simulink library "SUB_ECU_L4_MABX_HW_Interface"  (R2018a)
settings: Solver=VariableStepAuto  StartTime=0.0  StopTime=10.0  RelTol=1e-3
PostLoadFcn:
  | , if any(exist('dsrtsu_mdlpostloadfcn', 'file') == [2, 3, 6]), try dsrtsu_mdlpostloadfcn('Execute', bdroot); catch fprintf('Error in PostLoadFcn (dsrtsu_mdlpostloadfcn) for model "%s":\n %s\n', bdroot, lasterr); end, end,
undefined symbols (not defined in the file or in its folder): CANR_PROPB_REAX_3_13_CHANNEL_APV, CANR_PROPB_REAX_4_13_CHANNEL_APV, CANR_PROPB_XPR_1_50_CHANNEL_APV, ENUM_CAN_RX_T, ENUM_CAN_TX_T, ENUM_REAX_OPERATION_MODE_T, ENUM_SIGNAL_HEALTH_T, ENUM_XBR_CONTROL_MODE_T, ENUM_XBR_EBI_MODE_T, ENUM_XBR_PASS_THROUGH_ACTIVE_T, ENUM_XBR_PRIORITY_T, ENUM_XPR_INHIBIT_PARK_MANUAL_T, ENUM_XPR_INHIBIT_UNPARK_MANUAL_T, ENUM_XPR_PARK_MANUAL_T, ENUM_XPR_UNPARK_MANUAL_T, PROPB_REAX_1_E4_DES_POS_SIG_SRC_APV, PROPB_REAX_1_E4_DESIRED_OPMODE_APV, PROPB_REAX_1_E4_DESIRED_POSITION_APV, ptc_matlab_lib
libraries: PTC_MBDS_LIB x264, rtican x172, EmE_MBD_Blockset x39, simulink x34, $bdroot x16, rti1401lib_dio_type4 x8, simulink_need_slupdate x7, dsa_tcpip_lib x4, rti1401lib_adc_type4 x3, rtmapslib x3, rtitasklib x3
(part 45 of 51)

== system SUB_ECU_L4_MABX_HW_Interface/CAN_Out_PTC_1571/CAN_TX_1000ms/CAN_TX_AMB_00/TX_CAN4 ==
  Enable : Inport
  Data : Inport  Port=2
  AMB : rtican/RTICAN Transmit (TX)   Reserved1=[]  Reserved2=[]  Reserved3=[]  Reserved4=[]  SfcnMessage=[]  Msg_Struct=[]  BoardTypeNo=[]  BoardNo=[]  ChannelNo=[]  Parameters=[]  DialogFcn=[]  UnitName=[]  Revision=[]  UnitValues=[]  DSProperties=struct('RTI',struct('Version',uint32(5),'BlockType',struct('isSLSource',uint8(1),'isSLSink',uint8(1),'isHWSource',uint8(0),'isHWSink',uint8(0),'isSetup',uint8(0),'isInline',uint8(1),'isNonInline',uint8(0),'isInterrupt',uint8(0),'isChannelwise',uint8(0)),'IOBoardType','RTICAN','UnitType','MESSAGE','Identifier','TX','DialogType','MSVC','BlockSet','RTICAN','SlaveProcessor','CAN'))  RTIBlockInterface=struct('InputPortsWidth',int32([1 1 1 1 1]),'InputPortsActive',[1 1 1 1 1],'InputPortsName',{{'BarometricPress','CabInteriorTemp','AmbientAirTemp','EngAirIntakeTemp','RoadSurfaceTemp'}},'InputPortsDataType',{{'SS_DOUBLE','SS_DOUBLE','SS_DOUBLE','SS_DOUBLE','SS_DOUBLE'}},'OutputPortsWidth',int32([1 1 1 1]),'OutputPortsActive',[1 1 1 1],'OutputPortsName',{{['TX status'],['TX time'],['TX delta time'],['TX delay time']}},'DialogFcn','rtican_message_interface_gui','BlockDisplay',{{'','center'}},'IconTransparency','on','InitLevel',3,'BlockName',struct('Token',{{'AMB'}}),'SampleTime',{{-1}},'TriggerPort',{{'none'}},'EnablePort',{{'yes'}})  RTIBlockParameters="struct('BoardTypeNo',{{1,'OFF',[]}},'BoardNo',{{2,'ON',[1 16]}},'ChannelNo',{{2,'ON',[1 2]}},'Parameters',{{struct('DataFileSupport',struct('DataFileSelectedMaster',1,'DataFileSelectedLocal',0,'DataFileName',['c:\\data\\svn\\truck1571\\dbc\\mabx_can4.dbc|c:\\data\\svn\\svn\\powertrainsys\\trunk\\src\\projects_rcp\\my2017_rcp\\dbc files\\j1939.dbc|'],'DataFileDate',{{{['10-Feb-2017 15:17:28']},{['24-Aug-2017 12:01:59']}}},'SelectedFile',['<no file selected>']),'Options',struct('StatusSelected',1,'TimeSelected',1,'DeltaTimeSelected',1,'DelayTimeSelected',1,'DelayTimeTXCommandSelected',0,'EncodeSetUnusedBitsToOne',1,'EnableMsgLoopback',0,'TriggerPort',struct('Selected',0,'TriggerType',0),'EnablePortSelected',1,'SignalOnPortnameSelected',1,'UserCoding',struct('Selected',0,'InterfaceFile','UserEncodingFile','FcnName','UserEncodeFcn','InportSelected',0,'InportWidth',1,'OutportSelected',0,'OutportWidth',1),'TerminationMsg',struct('Selected',0,'Byte0_7','0'),'InitialMsg',struct('Selected',0,'Byte0_7','0')),'Message',struct('MsgOnBlocknameSelected',1,'MsgName','AMB','MsgIdFormat',1,'MsgId',419362048,'MsgLength',8,'NumSignals',5,'SampleTime',-1,'StartTime',struct('Selected',0,'Value',0),'AutoRepeatTime',struct('Selected',0,'Value',1),'Timeout',struct('Selected',0,'Value',0.1),'DelayTime',struct('Selected',0,'Value',0.1),'Signal',struct('SgnName',{'BarometricPress','CabInteriorTemp','AmbientAirTemp','EngAirIntakeTemp','RoadSurfaceTemp'},'SgnStartBit',{0,8,24,40,48},'SgnLength',{8,16,16,8,16},'SgnType',{0,0,0,0,0},'ModeValue',{-1,-1,-1,-1,-1},'DataType',{0,0,0,0,0},'ByteLayout',{0,0,0,0,0},'Factor',{2^-1,2^-5,2^-5,1,2^-5},'Offset',{0,-273,-273,-40,-273},'SgnComment',{{['Absolute air pressure of the atmosphere.']},{['Temperature of air inside the part of the vehicle that encloses the driver and vehicle operating controls.' char(10) '' char(10) 'Note: See also SPN 1691.  SPN 1662 is an additional diagnostic SPN associated with cab temperature.']},{['Temperature of air surrounding vehicle.']},{['Temperature of air entering vehicle air induction system.']},{['Indicated temperature of road surface over which vehicle is operating.']}},'SgnUnit',{'kPa','°C','°C','°C','°C'},'Min',{0,-273,-273,-40,-273},'Max',{125,1734.96875,1734.96875,210,1734.96875},'SLDataType',{'SS_DOUBLE','SS_DOUBLE','SS_DOUBLE','SS_DOUBLE','SS_DOUBLE'}),'MsgIdNumFormat',1,'MsgComment',{{['Ambient Conditions']}}),'Version',1.2,'general',struct('isFromLib',0)),'OFF',[]}},'GroupId',{{struct('Group',{{'RTICAN'}},'No',4,'Behavior',{{'NAMECHANGE'}},'BlockType',{{'SINK'}},'NameChangeFlag',0),'OFF',[]}},'SFcnRTICANMessage',{{struct('MsgType','TX','SFcnPortType','Scalar','MsgName','AMB','MsgIdFormat','XTD','MsgId',419362048,'MsgLength',8,'NumSignals',5,'SampleTime',-1,'StartTime',struct('Selected','no','Value',0),'AutoRepeatTime',struct('Selected','no','Value',1),'Timeout',struct('Selected','no','Value',0.1),'Signal',struct('SgnName',{'BarometricPress','CabInteriorTemp','AmbientAirTemp','EngAirIntakeTemp','RoadSurfaceTemp'},'SgnStartBit',{0,8,24,40,48},'SgnLength',{8,16,16,8,16},'SgnType',{'standard','standard','standard','standard','standard'},'ModeValue',{-1,-1,-1,-1,-1},'DataType',{['unsigned int'],['unsigned int'],['unsigned int'],['unsigned int'],['unsigned int']},'ByteLayout',{['little endian'],['little endian'],['little endian'],['little endian'],['little endian']},'Factor',{2^-1,2^-5,2^-5,1,2^-5},'Offset',{0,-273,-273,-40,-273},'SLDataType',{'SS_DOUBLE','SS_DOUBLE','SS_DOUBLE','SS_DOUBLE','SS_DOUBLE'}),'StatusSelected','yes','TimeSelected','yes','DeltaTimeSelected','yes','DelayTimeSelected','yes','DelayTimeTXCommandSelected','no','EncodeSetUnusedBitsToOne','yes','EnableMsgLoopback','no','TriggerPort',struct('Selected','no','TriggerType',0),'EnablePortSelected','yes','UserCoding',struct('Selected','no','InterfaceFile','UserEncodingFile','FcnName','UserEncodeFcn','InportSelected','no','InportWidth',1,'OutportSelected','no','OutportWidth',1),'TerminationMsg',struct('Selected','no','Byte0','0x00','Byte1','0x00','Byte2','0x00','Byte3','0x00','Byte4','0x00','Byte5','0x00','Byte6','0x00','Byte7','0x00'),'InitialMsg',struct('Selected','no','Byte0','0x00','Byte1','0x00','Byte2','0x00','Byte3','0x00','Byte4','0x00','Byte5','0x00','Byte6','0x00','Byte7','0x00'),'BoardType','DS1','BoardNo',2,'ControllerNo',2),'OFF',[]}},'TLCFileName',{{'rtican_tx_message','OFF',[]}})"  RTISFcnParameters=struct('SFcnRTICANMessage','struct','TLCFileName','char')  RTIBlockParaDefault=struct('BoardTypeNo',4302,'BoardNo',1,'ChannelNo',1,'Parameters',struct('DataFileSupport',struct('DataFileSelectedMaster',0,'DataFileSelectedLocal',0,'DataFileName','','DataFileDate','','SelectedFile',['<no file selected>']),'Options',struct('StatusSelected',1,'TimeSelected',1,'DeltaTimeSelected',1,'DelayTimeSelected',1,'DelayTimeTXCommandSelected',0,'EncodeSetUnusedBitsToOne',0,'EnableMsgLoopback',0,'TriggerPort',struct('Selected',0,'TriggerType','rising'),'EnablePortSelected',0,'SignalOnPortnameSelected',1,'UserCoding',struct('Selected',0,'InterfaceFile','UserEncodingFile','FcnName','UserEncodeFcn','InportSelected',0,'InportWidth',1,'OutportSelected',0,'OutportWidth',1),'TerminationMsg',struct('Selected',0,'Byte0_7','0'),'InitialMsg',struct('Selected',0,'Byte0_7','0')),'Message',struct('MsgOnBlocknameSelected',0,'MsgName',['TX Message'],'MsgIdFormat',0,'MsgId',100,'MsgLength',8,'NumSignals',1,'SampleTime',-1,'StartTime',struct('Selected',0,'Value',0),'AutoRepeatTime',struct('Selected',0,'Value',0.1),'Timeout',struct('Selected',0,'Value',0.1),'DelayTime',struct('Selected',0,'Value',0.1),'Signal',struct('SgnName',['TX signal'],'SgnStartBit',0,'SgnLength',8,'SgnType',0,'ModeValue',-1,'DataType',0,'SLDataType','SS_DOUBLE','ByteLayout',0,'Factor',1,'Offset',0,'Min',0,'Max',255,'SgnComment',{{}},'SgnUnit',''),'MsgIdNumFormat',0,'MsgComment',{{''}}),'Version',1.2,'general',struct('isFromLib',1)),'GroupId',struct('Group',{{'RTICAN'}},'No',1,'Behavior',{{'NAMECHANGE'}},'BlockType',{{'SINK'}},'NameChangeFlag',0),'SFcnRTICANMessage',struct('MsgType','TX','MsgName',['TX Message'],'MsgIdFormat','STD','MsgId',100,'MsgLength',2,'NumSignals',1,'SampleTime',-1,'StartTime',struct('Selected','no','Value',0),'AutoRepeatTime',struct('Selected','no','Value',0.1),'Timeout',struct('Selected','no','Value',0.1),'DelayTime',struct('Selected','no','Value',0.1),'Signal',struct('SgnName',['TX signal'],'SgnStartBit',0,'SgnLength',8,'SgnType','standard','ModeValue',-1,'DataType',['unsigned int'],'ByteLayout',['little endian'],'SLDataType','SS_DOUBLE','Factor',1,'Offset',0),'StatusSelected','yes','TimeSelected','yes','DeltaTimeSelected','yes','DelayTimeSelected','yes','EnablePortSelected','no','EnableMsgLoopback','no','DelayTimeTXCommandSelected','no','EncodeSetUnusedBitsToOne','no','UserCoding',struct('Selected','no','InterfaceFile','UserDecodingFile','FcnName','UserDecodeFcn','InportSelected','no','InportWidth',1,'OutportSelected','no','OutportWidth',1),'TerminationMsg',struct('Selected','no','Byte0','0x00','Byte1','0x00','Byte2','0x00','Byte3','0x00','Byte4','0x00','Byte5','0x00','Byte6','0x00','Byte7','0x00'),'InitialMsg',struct('Selected','no','Byte0','0x00','Byte1','0x00','Byte2','0x00','Byte3','0x00','Byte4','0x00','Byte5','0x00','Byte6','0x00','Byte7','0x00'),'TriggerPort',struct('Selected','no','TriggerType','rising'),'BoardType','DS4302','BoardNo',1,'ControllerNo',1,'SFcnPortType','Scalar'),'TLCFileName','rtican_tx_message')
      settings: AttributesFormatString=Group Id: RTICAN4\n  SourceProductName=dSPACE RTI CAN Blockset
  Bus Selector : BusSelector  OutputSignals=INPUTS.CAN.AMB_00.AMB_00Data.BarometricPress,INPUTS.CAN.AMB_00.AMB_00Data.CabInteriorTemp,INPUTS.CAN.AMB_00.AMB_00Data.AmbientAirTemp,INPUTS.CAN.AMB_00.AMB_00Data.EngAirIntakeTemp,INPUTS.CAN.AMB_00.AMB_00Data.RoadSurfaceTemp
  Terminator{,1..3} (4 alike) : Terminator
      settings: InitFcn=|
      | try
      |    MBDS_BlockCallback('Update', gcb);
      | end
  wires:
  Enable/1 -> AMB/Enable
  Data/1 -> Bus Selector/1
  AMB/2 -> Terminator1/1
  AMB/4 -> Terminator3/1
  AMB/3 -> Terminator2/1
  AMB/1 -> Terminator/1
  Bus Selector/1 -> AMB/1  "<BarometricPress>"
  Bus Selector/2 -> AMB/2  "<CabInteriorTemp>"
  Bus Selector/3 -> AMB/3  "<AmbientAirTemp>"
  Bus Selector/4 -> AMB/4  "<EngAirIntakeTemp>"
  Bus Selector/5 -> AMB/5  "<RoadSurfaceTemp>"

== system SUB_ECU_L4_MABX_HW_Interface/CAN_Out_PTC_1571/CAN_TX_100ms/CAN_TX_CCVS1_00/TX_CAN4 ==
  Enable : Inport
  Data : Inport  Port=2
  Bus Selector : BusSelector  OutputSignals=INPUTS.CAN.CCVS1_00.CCVS1Data.TwoSpeedAxleSwitch,INPUTS.CAN.CCVS1_00.CCVS1Data.ParkingBrakeSwitch,INPUTS.CAN.CCVS1_00.CCVS1Data.CruiseCtrlPauseSwitch,INPUTS.CAN.CCVS1_00.CCVS1Data.ParkBrakeReleaseInhibitRq,INPUTS.CAN.CCVS1_00.CCVS1Data.WheelBasedVehicleSpeed,INPUTS.CAN.CCVS1_00.CCVS1Data.CruiseCtrlActive,INPUTS.CAN.CCVS1_00.CCVS1Data.CruiseCtrlEnableSwitch,INPUTS.CAN.CCVS1_00.CCVS1Data.BrakeSwitch,INPUTS.CAN.CCVS1_00.CCVS1Data.ClutchSwitch,INPUTS.CAN.CCVS1_00.CCVS1Data.CruiseCtrlSetSwitch,INPUTS.CAN.CCVS1_00.CCVS1Data.CruiseCtrlCoastSwitch,INPUTS.CAN.CCVS1_00.CCVS1Data.CruiseCtrlResumeSwitch,INPUTS.CAN.CCVS1_00.CCVS1Data.CruiseCtrlAccelerateSwitch,INPUTS.CAN.CCVS1_00.CCVS1Data.CruiseCtrlSetSpeed,INPUTS.CAN.CCVS1_00.CCVS1Data.PTOGovernorState,INPUTS.CAN.CCVS1_00.CCVS1Data.CruiseCtrlStates,INPUTS.CAN.CCVS1_00.CCVS1Data.EngIdleIncrementSwitch,INPUTS.CAN.CCVS1_00.CCVS1Data.EngIdleDecrementSwitch,INPUTS.CAN.CCVS1_00.CCVS1Data.EngTestModeSwitch,INPUTS.CAN.CCVS1_00.CCVS1Data.EngShutdownOverrideSwitch
  CCVS1_00 : rtican/RTICAN Transmit (TX)   Reserved1=[]  Reserved2=[]  Reserved3=[]  Reserved4=[]  SfcnMessage=[]  Msg_Struct=[]  BoardTypeNo=[]  BoardNo=[]  ChannelNo=[]  Parameters=[]  DialogFcn=[]  UnitName=[]  Revision=[]  UnitValues=[]  DSProperties=struct('RTI',struct('Version',uint32(5),'BlockType',struct('isSLSource',uint8(1),'isSLSink',uint8(1),'isHWSource',uint8(0),'isHWSink',uint8(0),'isSetup',uint8(0),'isInline',uint8(1),'isNonInline',uint8(0),'isInterrupt',uint8(0),'isChannelwise',uint8(0)),'IOBoardType','RTICAN','UnitType','MESSAGE','Identifier','TX','DialogType','MSVC','BlockSet','RTICAN','SlaveProcessor','CAN'))  RTIBlockInterface=struct('InputPortsWidth',int32([1 1 1 1 1 1 1 1 1 1 1 1 1 1 1 1 1 1 1 1]),'InputPortsActive',ones(1,20),'InputPortsName',{{'TwoSpeedAxleSwitch','ParkingBrakeSwitch','CruiseCtrlPauseSwitch','ParkBrakeReleaseInhibitRq','WheelBasedVehicleSpeed','CruiseCtrlActive','CruiseCtrlEnableSwitch','BrakeSwitch','ClutchSwitch','CruiseCtrlSetSwitch','CruiseCtrlCoastSwitch','CruiseCtrlResumeSwitch','CruiseCtrlAccelerateSwitch','CruiseCtrlSetSpeed','PTOGovernorState','CruiseCtrlStates','EngIdleIncrementSwitch','EngIdleDecrementSwitch','EngTestModeSwitch','EngShutdownOverrideSwitch'}},'InputPortsDataType',{{'SS_DOUBLE','SS_DOUBLE','SS_DOUBLE','SS_DOUBLE','SS_DOUBLE','SS_DOUBLE','SS_DOUBLE','SS_DOUBLE','SS_DOUBLE','SS_DOUBLE','SS_DOUBLE','SS_DOUBLE','SS_DOUBLE','SS_DOUBLE','SS_DOUBLE','SS_DOUBLE','SS_DOUBLE','SS_DOUBLE','SS_DOUBLE','SS_DOUBLE'}},'OutputPortsWidth',int32([1 1 1 1]),'OutputPortsActive',[1 1 1 1],'OutputPortsName',{{['TX status'],['TX time'],['TX delta time'],['TX delay time']}},'DialogFcn','rtican_message_interface_gui','BlockDisplay',{{'','center'}},'IconTransparency','on','InitLevel',3,'BlockName',struct('Token',{{'CCVS1_00'}}),'SampleTime',{{-1}},'TriggerPort',{{'none'}},'EnablePort',{{'yes'}})  RTIBlockParameters=struct('BoardTypeNo',{{1,'OFF',[]}},'BoardNo',{{2,'ON',[1 16]}},'ChannelNo',{{2,'ON',[1 2]}},'Parameters',{{struct('DataFileSupport',struct('DataFileSelectedMaster',1,'DataFileSelectedLocal',0,'DataFileName',['c:\data\svn\truck1571\dbc\mabx_can4.dbc|c:\data\svn\svn\powertrainsys\trunk\src\projects_rcp\my2017_rcp\dbc files\j1939.dbc|'],'DataFileDate',{{{['11-Jan-2017 09:37:25']}}},'SelectedFile',['<no file selected>']),'Options',struct('StatusSelected',1,'TimeSelected',1,'DeltaTimeSelected',1,'DelayTimeSelected',1,'DelayTimeTXCommandSelected',0,'EncodeSetUnusedBitsToOne',1,'EnableMsgLoopback',0,'TriggerPort',struct('Selected',0,'TriggerType',0),'EnablePortSelected',1,'SignalOnPortnameSelected',1,'UserCoding',struct('Selected',0,'InterfaceFile','UserEncodingFile','FcnName','UserEncodeFcn','InportSelected',0,'InportWidth',1,'OutportSelected',0,'OutportWidth',1),'TerminationMsg',struct('Selected',0,'Byte0_7','0'),'InitialMsg',struct('Selected',0,'Byte0_7','0')),'Message',struct('MsgOnBlocknameSelected',1,'MsgName','CCVS1_00','MsgIdFormat',1,'MsgId',419361024,'MsgLength',8,'NumSignals',20,'SampleTime',-1,'StartTime',struct('Selected',0,'Value',0),'AutoRepeatTime',struct('Selected',0,'Value',0.1),'Timeout',struct('Selected',0,'Value',0.1),'DelayTime',struct('Selected',0,'Value',0.1),'Signal',struct('SgnName',{'TwoSpeedAxleSwitch','ParkingBrakeSwitch','CruiseCtrlPauseSwitch','ParkBrakeReleaseInhibitRq','WheelBasedVehicleSpeed','CruiseCtrlActive','CruiseCtrlEnableSwitch','BrakeSwitch','ClutchSwitch','CruiseCtrlSetSwitch','CruiseCtrlCoastSwitch','CruiseCtrlResumeSwitch','CruiseCtrlAccelerateSwitch','CruiseCtrlSetSpeed','PTOGovernorState','CruiseCtrlStates','EngIdleIncrementSwitch','EngIdleDecrementSwitch','EngTestModeSwitch','EngShutdownOverrideSwitch'},'SgnStartBit',{0,2,4,6,8,24,26,28,30,32,34,36,38,40,48,53,56,58,60,62},'SgnLength',{2,2,2,2,16,2,2,2,2,2,2,2,2,8,5,3,2,2,2,2},'SgnType',{0,0,0,0,0,0,0,0,0,0,0,0,0,0,0,0,0,0,0,0},'ModeValue',{-1,-1,-1,-1,-1,-1,-1,-1,-1,-1,-1,-1,-1,-1,-1,-1,-1,-1,-1,-1},'DataType',{0,0,0,0,0,0,0,0,0,0,0,0,0,0,0,0,0,0,0,0},'ByteLayout',{0,0,0,0,0,0,0,0,0,0,0,0,0,0,0,0,0,0,0,0},'Factor',{1,1,1,1,2^-8,1,1,1,1,1,1,1,1,1,1,1,1,1,1,1},'Offset',{0,0,0,0,0,0,0,0,0,0,0,0,0,0,0,0,0,0,0,0},'SgnComment',{{['Switch signal which indicates the current axle range.']},{['Switch signal which indicates when the parking brake is set.']},{['Switch signal which indicates the position of the Cruise Control Pause Switch used on Remote Cruise Control applications.']},{['Park Brake Release Inhibit Request signals the desire that an applied park brake remain applied and limit the ability of the']},{['Speed of the vehicle as calculated from wheel or tailshaft speed.']},{['Cruise control is switched on.']},{['Switch signal which indicates that it is possible to manage the cruise control function.']},{['Switch signal which indicates that the driver operated brake foot pedal is being pressed.']},{['Switch signal which indicates that the clutch pedal is being pressed.']},{['Switch signal of the cruise control activator which indicates that the activator is in the position “set.']},{['Switch signal of the cruise control activator which indicates that the activator is in the position “coast (decelerate).']},{['Switch signal of the cruise control activator which indicates that the activator is in the position “resume.']},{['Switch signal of the cruise control activator which indicates that the activator is in the position “accelerate.']},{['Value of set (chosen) velocity of velocity control system.']},{['This parameter is used to indicate the current state or mode of operation by the power takeoff (PTO) governor.']},{['This parameter is used to indicate the current state, or mode, of operation by the cruise control device.']},{['Switch signal which indicates the position of the idle increment switch.']},{['Switch signal which indicates the position of the idle decrement switch.']},{['Switch signal which indicates the position of the engine test mode switch.']},{['Switch signal which indicates the position of the engine shutdown override switch.']}},'SgnUnit',{'','','','','km/h','','','','','','','','','km/h','','','','','',''},'Min',{0,0,0,0,0,0,0,0,0,0,0,0,0,0,0,0,0,0,0,0},'Max',{3,3,3,3,250.996,3,3,3,3,3,3,3,3,250,31,7,3,3,3,3},'SLDataType',{'SS_DOUBLE','SS_DOUBLE','SS_DOUBLE','SS_DOUBLE','SS_DOUBLE','SS_DOUBLE','SS_DOUBLE','SS_DOUBLE','SS_DOUBLE','SS_DOUBLE','SS_DOUBLE','SS_DOUBLE','SS_DOUBLE','SS_DOUBLE','SS_DOUBLE','SS_DOUBLE','SS_DOUBLE','SS_DOUBLE','SS_DOUBLE','SS_DOUBLE'}),'MsgIdNumFormat',1,'MsgComment',{{['Cruise Control/Vehicle Speed']}}),'Version',1.2,'general',struct('isFromLib',0)),'OFF',[]}},'GroupId',{{struct('Group',{{'RTICAN'}},'No',4,'Behavior',{{'NAMECHANGE'}},'BlockType',{{'SINK'}},'NameChangeFlag',0),'OFF',[]}},'SFcnRTICANMessage',{{struct('MsgType','TX','SFcnPortType','Scalar','MsgName','CCVS1_00','MsgIdFormat','XTD','MsgId',419361024,'MsgLength',8,'NumSignals',20,'SampleTime',-1,'StartTime',struct('Selected','no','Value',0),'AutoRepeatTime',struct('Selected','no','Value',0.1),'Timeout',struct('Selected','no','Value',0.1),'Signal',struct('SgnName',{'TwoSpeedAxleSwitch','ParkingBrakeSwitch','CruiseCtrlPauseSwitch','ParkBrakeReleaseInhibitRq','WheelBasedVehicleSpeed','CruiseCtrlActive','CruiseCtrlEnableSwitch','BrakeSwitch','ClutchSwitch','CruiseCtrlSetSwitch','CruiseCtrlCoastSwitch','CruiseCtrlResumeSwitch','CruiseCtrlAccelerateSwitch','CruiseCtrlSetSpeed','PTOGovernorState','CruiseCtrlStates','EngIdleIncrementSwitch','EngIdleDecrementSwitch','EngTestModeSwitch','EngShutdownOverrideSwitch'},'SgnStartBit',{0,2,4,6,8,24,26,28,30,32,34,36,38,40,48,53,56,58,60,62},'SgnLength',{2,2,2,2,16,2,2,2,2,2,2,2,2,8,5,3,2,2,2,2},'SgnType',{'standard','standard','standard','standard','standard','standard','standard','standard','standard','standard','standard','standard','standard','standard','standard','standard','standard','standard','standard','standard'},'ModeValue',{-1,-1,-1,-1,-1,-1,-1,-1,-1,-1,-1,-1,-1,-1,-1,-1,-1,-1,-1,-1},'DataType',{['unsigned int'],['unsigned int'],['unsigned int'],['unsigned int'],['unsigned int'],['unsigned int'],['unsigned int'],['unsigned int'],['unsigned int'],['unsigned int'],['unsigned int'],['unsigned int'],['unsigned int'],['unsigned int'],['unsigned int'],['unsigned int'],['unsigned int'],['unsigned int'],['unsigned int'],['unsigned int']},'ByteLayout',{['little endian'],['little endian'],['little endian'],['little endian'],['little endian'],['little endian'],['little endian'],['little endian'],['little endian'],['little endian'],['little endian'],['little endian'],['little endian'],['little endian'],['little endian'],['little endian'],['little endian'],['little endian'],['little endian'],['little endian']},'Factor',{1,1,1,1,2^-8,1,1,1,1,1,1,1,1,1,1,1,1,1,1,1},'Offset',{0,0,0,0,0,0,0,0,0,0,0,0,0,0,0,0,0,0,0,0},'SLDataType',{'SS_DOUBLE','SS_DOUBLE','SS_DOUBLE','SS_DOUBLE','SS_DOUBLE','SS_DOUBLE','SS_DOUBLE','SS_DOUBLE','SS_DOUBLE','SS_DOUBLE','SS_DOUBLE','SS_DOUBLE','SS_DOUBLE','SS_DOUBLE','SS_DOUBLE','SS_DOUBLE','SS_DOUBLE','SS_DOUBLE','SS_DOUBLE','SS_DOUBLE'}),'StatusSelected','yes','TimeSelected','yes','DeltaTimeSelected','yes','DelayTimeSelected','yes','DelayTimeTXCommandSelected','no','EncodeSetUnusedBitsToOne','yes','EnableMsgLoopback','no','TriggerPort',struct('Selected','no','TriggerType',0),'EnablePortSelected','yes','UserCoding',struct('Selected','no','InterfaceFile','UserEncodingFile','FcnName','UserEncodeFcn','InportSelected','no','InportWidth',1,'OutportSelected','no','OutportWidth',1),'TerminationMsg',struct('Selected','no','Byte0','0x00','Byte1','0x00','Byte2','0x00','Byte3','0x00','Byte4','0x00','Byte5','0x00','Byte6','0x00','Byte7','0x00'),'InitialMsg',struct('Selected','no','Byte0','0x00','Byte1','0x00','Byte2','0x00','Byte3','0x00','Byte4','0x00','Byte5','0x00','Byte6','0x00','Byte7','0x00'),'BoardType','DS1','BoardNo',2,'ControllerNo',2),'OFF',[]}},'TLCFileName',{{'rtican_tx_message','OFF',[]}})  RTISFcnParameters=struct('SFcnRTICANMessage','struct','TLCFileName','char')  RTIBlockParaDefault=struct('BoardTypeNo',4302,'BoardNo',1,'ChannelNo',1,'Parameters',struct('DataFileSupport',struct('DataFileSelectedMaster',0,'DataFileSelectedLocal',0,'DataFileName','','DataFileDate','','SelectedFile',['<no file selected>']),'Options',struct('StatusSelected',1,'TimeSelected',1,'DeltaTimeSelected',1,'DelayTimeSelected',1,'DelayTimeTXCommandSelected',0,'EncodeSetUnusedBitsToOne',0,'EnableMsgLoopback',0,'TriggerPort',struct('Selected',0,'TriggerType','rising'),'EnablePortSelected',0,'SignalOnPortnameSelected',1,'UserCoding',struct('Selected',0,'InterfaceFile','UserEncodingFile','FcnName','UserEncodeFcn','InportSelected',0,'InportWidth',1,'OutportSelected',0,'OutportWidth',1),'TerminationMsg',struct('Selected',0,'Byte0_7','0'),'InitialMsg',struct('Selected',0,'Byte0_7','0')),'Message',struct('MsgOnBlocknameSelected',0,'MsgName',['TX Message'],'MsgIdFormat',0,'MsgId',100,'MsgLength',8,'NumSignals',1,'SampleTime',-1,'StartTime',struct('Selected',0,'Value',0),'AutoRepeatTime',struct('Selected',0,'Value',0.1),'Timeout',struct('Selected',0,'Value',0.1),'DelayTime',struct('Selected',0,'Value',0.1),'Signal',struct('SgnName',['TX signal'],'SgnStartBit',0,'SgnLength',8,'SgnType',0,'ModeValue',-1,'DataType',0,'SLDataType','SS_DOUBLE','ByteLayout',0,'Factor',1,'Offset',0,'Min',0,'Max',255,'SgnComment',{{}},'SgnUnit',''),'MsgIdNumFormat',0,'MsgComment',{{''}}),'Version',1.2,'general',struct('isFromLib',1)),'GroupId',struct('Group',{{'RTICAN'}},'No',1,'Behavior',{{'NAMECHANGE'}},'BlockType',{{'SINK'}},'NameChangeFlag',0),'SFcnRTICANMessage',struct('MsgType','TX','MsgName',['TX Message'],'MsgIdFormat','STD','MsgId',100,'MsgLength',2,'NumSignals',1,'SampleTime',-1,'StartTime',struct('Selected','no','Value',0),'AutoRepeatTime',struct('Selected','no','Value',0.1),'Timeout',struct('Selected','no','Value',0.1),'DelayTime',struct('Selected','no','Value',0.1),'Signal',struct('SgnName',['TX signal'],'SgnStartBit',0,'SgnLength',8,'SgnType','standard','ModeValue',-1,'DataType',['unsigned int'],'ByteLayout',['little endian'],'SLDataType','SS_DOUBLE','Factor',1,'Offset',0),'StatusSelected','yes','TimeSelected','yes','DeltaTimeSelected','yes','DelayTimeSelected','yes','EnablePortSelected','no','EnableMsgLoopback','no','DelayTimeTXCommandSelected','no','EncodeSetUnusedBitsToOne','no','UserCoding',struct('Selected','no','InterfaceFile','UserDecodingFile','FcnName','UserDecodeFcn','InportSelected','no','InportWidth',1,'OutportSelected','no','OutportWidth',1),'TerminationMsg',struct('Selected','no','Byte0','0x00','Byte1','0x00','Byte2','0x00','Byte3','0x00','Byte4','0x00','Byte5','0x00','Byte6','0x00','Byte7','0x00'),'InitialMsg',struct('Selected','no','Byte0','0x00','Byte1','0x00','Byte2','0x00','Byte3','0x00','Byte4','0x00','Byte5','0x00','Byte6','0x00','Byte7','0x00'),'TriggerPort',struct('Selected','no','TriggerType','rising'),'BoardType','DS4302','BoardNo',1,'ControllerNo',1,'SFcnPortType','Scalar'),'TLCFileName','rtican_tx_message')
      settings: AttributesFormatString=Group Id: RTICAN4\n  SourceProductName=dSPACE RTI CAN Blockset
  Terminator{,1..3} (4 alike) : Terminator
      settings: InitFcn=|
      | try
      |    MBDS_BlockCallback('Update', gcb);
      | end
  wires:
  Data/1 -> Bus Selector/1
  CCVS1_00/2 -> Terminator1/1
  CCVS1_00/4 -> Terminator3/1
  CCVS1_00/3 -> Terminator2/1
  CCVS1_00/1 -> Terminator/1
  Enable/1 -> CCVS1_00/Enable
  Bus Selector/1 -> CCVS1_00/1  "<TwoSpeedAxleSwitch>"
  Bus Selector/15 -> CCVS1_00/15  "<PTOGovernorState>"
  Bus Selector/19 -> CCVS1_00/19  "<EngTestModeSwitch>"
  Bus Selector/12 -> CCVS1_00/12  "<CruiseCtrlResumeSwitch>"
  Bus Selector/18 -> CCVS1_00/18  "<EngIdleDecrementSwitch>"
  Bus Selector/9 -> CCVS1_00/9  "<ClutchSwitch>"
  Bus Selector/7 -> CCVS1_00/7  "<CruiseCtrlEnableSwitch>"
  Bus Selector/10 -> CCVS1_00/10  "<CruiseCtrlSetSwitch>"
  Bus Selector/13 -> CCVS1_00/13  "<CruiseCtrlAccelerateSwitch>"
  Bus Selector/8 -> CCVS1_00/8  "<BrakeSwitch>"
  Bus Selector/5 -> CCVS1_00/5  "<WheelBasedVehicleSpeed>"
  Bus Selector/16 -> CCVS1_00/16  "<CruiseCtrlStates>"
  Bus Selector/2 -> CCVS1_00/2  "<ParkingBrakeSwitch>"
  Bus Selector/3 -> CCVS1_00/3  "<CruiseCtrlPauseSwitch>"
  Bus Selector/11 -> CCVS1_00/11  "<CruiseCtrlCoastSwitch>"
  Bus Selector/14 -> CCVS1_00/14  "<CruiseCtrlSetSpeed>"
  Bus Selector/6 -> CCVS1_00/6  "<CruiseCtrlActive>"
  Bus Selector/4 -> CCVS1_00/4  "<ParkBrakeReleaseInhibitRq>"
  Bus Selector/20 -> CCVS1_00/20  "<EngShutdownOverrideSwitch>"
  Bus Selector/17 -> CCVS1_00/17  "<EngIdleIncrementSwitch>"

== system SUB_ECU_L4_MABX_HW_Interface/CAN_Out_PTC_1571/CAN_TX_100ms/CAN_TX_CCVS1_00/TX_CAN5 ==
  note: Gateway of Vehicle Speed to REAX system
  Enable : Inport
  Data : Inport  Port=2
  Bus Selector : BusSelector  OutputSignals=INPUTS.CAN.CCVS1_00.CCVS1Data.TwoSpeedAxleSwitch,INPUTS.CAN.CCVS1_00.CCVS1Data.ParkingBrakeSwitch,INPUTS.CAN.CCVS1_00.CCVS1Data.CruiseCtrlPauseSwitch,INPUTS.CAN.CCVS1_00.CCVS1Data.ParkBrakeReleaseInhibitRq,INPUTS.CAN.CCVS1_00.CCVS1Data.WheelBasedVehicleSpeed,INPUTS.CAN.CCVS1_00.CCVS1Data.CruiseCtrlActive,INPUTS.CAN.CCVS1_00.CCVS1Data.CruiseCtrlEnableSwitch,INPUTS.CAN.CCVS1_00.CCVS1Data.BrakeSwitch,INPUTS.CAN.CCVS1_00.CCVS1Data.ClutchSwitch,INPUTS.CAN.CCVS1_00.CCVS1Data.CruiseCtrlSetSwitch,INPUTS.CAN.CCVS1_00.CCVS1Data.CruiseCtrlCoastSwitch,INPUTS.CAN.CCVS1_00.CCVS1Data.CruiseCtrlResumeSwitch,INPUTS.CAN.CCVS1_00.CCVS1Data.CruiseCtrlAccelerateSwitch,INPUTS.CAN.CCVS1_00.CCVS1Data.CruiseCtrlSetSpeed,INPUTS.CAN.CCVS1_00.CCVS1Data.PTOGovernorState,INPUTS.CAN.CCVS1_00.CCVS1Data.CruiseCtrlStates,INPUTS.CAN.CCVS1_00.CCVS1Data.EngIdleIncrementSwitch,INPUTS.CAN.CCVS1_00.CCVS1Data.EngIdleDecrementSwitch,INPUTS.CAN.CCVS1_00.CCVS1Data.EngTestModeSwitch,INPUTS.CAN.CCVS1_00.CCVS1Data.EngShutdownOverrideSwitch
  CCVS1_00 : rtican/RTICAN Transmit (TX)   Reserved1=[]  Reserved2=[]  Reserved3=[]  Reserved4=[]  SfcnMessage=[]  Msg_Struct=[]  BoardTypeNo=[]  BoardNo=[]  ChannelNo=[]  Parameters=[]  DialogFcn=[]  UnitName=[]  Revision=[]  UnitValues=[]  DSProperties=struct('RTI',struct('Version',uint32(5),'BlockType',struct('isSLSource',uint8(1),'isSLSink',uint8(1),'isHWSource',uint8(0),'isHWSink',uint8(0),'isSetup',uint8(0),'isInline',uint8(1),'isNonInline',uint8(0),'isInterrupt',uint8(0),'isChannelwise',uint8(0)),'IOBoardType','RTICAN','UnitType','MESSAGE','Identifier','TX','DialogType','MSVC','BlockSet','RTICAN','SlaveProcessor','CAN'))  RTIBlockInterface=struct('InputPortsWidth',int32([1 1 1 1 1 1 1 1 1 1 1 1 1 1 1 1 1 1 1 1]),'InputPortsActive',ones(1,20),'InputPortsName',{{'TwoSpeedAxleSwitch','ParkingBrakeSwitch','CruiseCtrlPauseSwitch','ParkBrakeReleaseInhibitRq','WheelBasedVehicleSpeed','CruiseCtrlActive','CruiseCtrlEnableSwitch','BrakeSwitch','ClutchSwitch','CruiseCtrlSetSwitch','CruiseCtrlCoastSwitch','CruiseCtrlResumeSwitch','CruiseCtrlAccelerateSwitch','CruiseCtrlSetSpeed','PTOGovernorState','CruiseCtrlStates','EngIdleIncrementSwitch','EngIdleDecrementSwitch','EngTestModeSwitch','EngShutdownOverrideSwitch'}},'InputPortsDataType',{{'SS_DOUBLE','SS_DOUBLE','SS_DOUBLE','SS_DOUBLE','SS_DOUBLE','SS_DOUBLE','SS_DOUBLE','SS_DOUBLE','SS_DOUBLE','SS_DOUBLE','SS_DOUBLE','SS_DOUBLE','SS_DOUBLE','SS_DOUBLE','SS_DOUBLE','SS_DOUBLE','SS_DOUBLE','SS_DOUBLE','SS_DOUBLE','SS_DOUBLE'}},'OutputPortsWidth',int32([1 1 1 1]),'OutputPortsActive',[1 1 1 1],'OutputPortsName',{{['TX status'],['TX time'],['TX delta time'],['TX delay time']}},'DialogFcn','rtican_message_interface_gui','BlockDisplay',{{'','center'}},'IconTransparency','on','InitLevel',3,'BlockName',struct('Token',{{'CCVS1_00'}}),'SampleTime',{{-1}},'TriggerPort',{{'none'}},'EnablePort',{{'yes'}})  RTIBlockParameters=struct('BoardTypeNo',{{1,'OFF',[]}},'BoardNo',{{3,'ON',[1 16]}},'ChannelNo',{{1,'ON',[1 2]}},'Parameters',{{struct('DataFileSupport',struct('DataFileSelectedMaster',1,'DataFileSelectedLocal',0,'DataFileName','c:\data\svn\truck1571\dbc\mabx_can4_chrisbaltonallstandard.dbc|c:\data\svn\truck1571\dbc\mabx_can4.dbc|','DataFileDate',{{{['11-Jan-2017 09:37:25']}}},'SelectedFile',['<no file selected>']),'Options',struct('StatusSelected',1,'TimeSelected',1,'DeltaTimeSelected',1,'DelayTimeSelected',1,'DelayTimeTXCommandSelected',0,'EncodeSetUnusedBitsToOne',0,'EnableMsgLoopback',0,'TriggerPort',struct('Selected',0,'TriggerType',0),'EnablePortSelected',1,'SignalOnPortnameSelected',1,'UserCoding',struct('Selected',0,'InterfaceFile','UserEncodingFile','FcnName','UserEncodeFcn','InportSelected',0,'InportWidth',1,'OutportSelected',0,'OutportWidth',1),'TerminationMsg',struct('Selected',0,'Byte0_7','0'),'InitialMsg',struct('Selected',0,'Byte0_7','0')),'Message',struct('MsgOnBlocknameSelected',1,'MsgName','CCVS1_00','MsgIdFormat',1,'MsgId',218034432,'MsgLength',8,'NumSignals',20,'SampleTime',-1,'StartTime',struct('Selected',0,'Value',0),'AutoRepeatTime',struct('Selected',0,'Value',0.1),'Timeout',struct('Selected',0,'Value',0.1),'DelayTime',struct('Selected',0,'Value',0.1),'Signal',struct('SgnName',{'TwoSpeedAxleSwitch','ParkingBrakeSwitch','CruiseCtrlPauseSwitch','ParkBrakeReleaseInhibitRq','WheelBasedVehicleSpeed','CruiseCtrlActive','CruiseCtrlEnableSwitch','BrakeSwitch','ClutchSwitch','CruiseCtrlSetSwitch','CruiseCtrlCoastSwitch','CruiseCtrlResumeSwitch','CruiseCtrlAccelerateSwitch','CruiseCtrlSetSpeed','PTOGovernorState','CruiseCtrlStates','EngIdleIncrementSwitch','EngIdleDecrementSwitch','EngTestModeSwitch','EngShutdownOverrideSwitch'},'SgnStartBit',{0,2,4,6,8,24,26,28,30,32,34,36,38,40,48,53,56,58,60,62},'SgnLength',{2,2,2,2,16,2,2,2,2,2,2,2,2,8,5,3,2,2,2,2},'SgnType',{0,0,0,0,0,0,0,0,0,0,0,0,0,0,0,0,0,0,0,0},'ModeValue',{-1,-1,-1,-1,-1,-1,-1,-1,-1,-1,-1,-1,-1,-1,-1,-1,-1,-1,-1,-1},'DataType',{0,0,0,0,0,0,0,0,0,0,0,0,0,0,0,0,0,0,0,0},'ByteLayout',{0,0,0,0,0,0,0,0,0,0,0,0,0,0,0,0,0,0,0,0},'Factor',{1,1,1,1,2^-8,1,1,1,1,1,1,1,1,1,1,1,1,1,1,1},'Offset',{0,0,0,0,0,0,0,0,0,0,0,0,0,0,0,0,0,0,0,0},'SgnComment',{{['Switch signal which indicates the current axle range.']},{['Switch signal which indicates when the parking brake is set.']},{['Switch signal which indicates the position of the Cruise Control Pause Switch used on Remote Cruise Control applications.']},{['Park Brake Release Inhibit Request signals the desire that an applied park brake remain applied and limit the ability of the']},{['Speed of the vehicle as calculated from wheel or tailshaft speed.']},{['Cruise control is switched on.']},{['Switch signal which indicates that it is possible to manage the cruise control function.']},{['Switch signal which indicates that the driver operated brake foot pedal is being pressed.']},{['Switch signal which indicates that the clutch pedal is being pressed.']},{['Switch signal of the cruise control activator which indicates that the activator is in the position “set.']},{['Switch signal of the cruise control activator which indicates that the activator is in the position “coast (decelerate).']},{['Switch signal of the cruise control activator which indicates that the activator is in the position “resume.']},{['Switch signal of the cruise control activator which indicates that the activator is in the position “accelerate.']},{['Value of set (chosen) velocity of velocity control system.']},{['This parameter is used to indicate the current state or mode of operation by the power takeoff (PTO) governor.']},{['This parameter is used to indicate the current state, or mode, of operation by the cruise control device.']},{['Switch signal which indicates the position of the idle increment switch.']},{['Switch signal which indicates the position of the idle decrement switch.']},{['Switch signal which indicates the position of the engine test mode switch.']},{['Switch signal which indicates the position of the engine shutdown override switch.']}},'SgnUnit',{'','','','','km/h','','','','','','','','','km/h','','','','','',''},'Min',{0,0,0,0,0,0,0,0,0,0,0,0,0,0,0,0,0,0,0,0},'Max',{3,3,3,3,250.996,3,3,3,3,3,3,3,3,250,31,7,3,3,3,3},'SLDataType',{'SS_DOUBLE','SS_DOUBLE','SS_DOUBLE','SS_DOUBLE','SS_DOUBLE','SS_DOUBLE','SS_DOUBLE','SS_DOUBLE','SS_DOUBLE','SS_DOUBLE','SS_DOUBLE','SS_DOUBLE','SS_DOUBLE','SS_DOUBLE','SS_DOUBLE','SS_DOUBLE','SS_DOUBLE','SS_DOUBLE','SS_DOUBLE','SS_DOUBLE'}),'MsgIdNumFormat',0,'MsgComment',{{['Cruise Control/Vehicle Speed']}}),'Version',1.2,'general',struct('isFromLib',0)),'OFF',[]}},'GroupId',{{struct('Group',{{'RTICAN'}},'No',5,'Behavior',{{'NAMECHANGE'}},'BlockType',{{'SINK'}},'NameChangeFlag',0),'OFF',[]}},'SFcnRTICANMessage',{{struct('MsgType','TX','SFcnPortType','Scalar','MsgName','CCVS1_00','MsgIdFormat','XTD','MsgId',218034432,'MsgLength',8,'NumSignals',20,'SampleTime',-1,'StartTime',struct('Selected','no','Value',0),'AutoRepeatTime',struct('Selected','no','Value',0.1),'Timeout',struct('Selected','no','Value',0.1),'Signal',struct('SgnName',{'TwoSpeedAxleSwitch','ParkingBrakeSwitch','CruiseCtrlPauseSwitch','ParkBrakeReleaseInhibitRq','WheelBasedVehicleSpeed','CruiseCtrlActive','CruiseCtrlEnableSwitch','BrakeSwitch','ClutchSwitch','CruiseCtrlSetSwitch','CruiseCtrlCoastSwitch','CruiseCtrlResumeSwitch','CruiseCtrlAccelerateSwitch','CruiseCtrlSetSpeed','PTOGovernorState','CruiseCtrlStates','EngIdleIncrementSwitch','EngIdleDecrementSwitch','EngTestModeSwitch','EngShutdownOverrideSwitch'},'SgnStartBit',{0,2,4,6,8,24,26,28,30,32,34,36,38,40,48,53,56,58,60,62},'SgnLength',{2,2,2,2,16,2,2,2,2,2,2,2,2,8,5,3,2,2,2,2},'SgnType',{'standard','standard','standard','standard','standard','standard','standard','standard','standard','standard','standard','standard','standard','standard','standard','standard','standard','standard','standard','standard'},'ModeValue',{-1,-1,-1,-1,-1,-1,-1,-1,-1,-1,-1,-1,-1,-1,-1,-1,-1,-1,-1,-1},'DataType',{['unsigned int'],['unsigned int'],['unsigned int'],['unsigned int'],['unsigned int'],['unsigned int'],['unsigned int'],['unsigned int'],['unsigned int'],['unsigned int'],['unsigned int'],['unsigned int'],['unsigned int'],['unsigned int'],['unsigned int'],['unsigned int'],['unsigned int'],['unsigned int'],['unsigned int'],['unsigned int']},'ByteLayout',{['little endian'],['little endian'],['little endian'],['little endian'],['little endian'],['little endian'],['little endian'],['little endian'],['little endian'],['little endian'],['little endian'],['little endian'],['little endian'],['little endian'],['little endian'],['little endian'],['little endian'],['little endian'],['little endian'],['little endian']},'Factor',{1,1,1,1,2^-8,1,1,1,1,1,1,1,1,1,1,1,1,1,1,1},'Offset',{0,0,0,0,0,0,0,0,0,0,0,0,0,0,0,0,0,0,0,0},'SLDataType',{'SS_DOUBLE','SS_DOUBLE','SS_DOUBLE','SS_DOUBLE','SS_DOUBLE','SS_DOUBLE','SS_DOUBLE','SS_DOUBLE','SS_DOUBLE','SS_DOUBLE','SS_DOUBLE','SS_DOUBLE','SS_DOUBLE','SS_DOUBLE','SS_DOUBLE','SS_DOUBLE','SS_DOUBLE','SS_DOUBLE','SS_DOUBLE','SS_DOUBLE'}),'StatusSelected','yes','TimeSelected','yes','DeltaTimeSelected','yes','DelayTimeSelected','yes','DelayTimeTXCommandSelected','no','EncodeSetUnusedBitsToOne','no','EnableMsgLoopback','no','TriggerPort',struct('Selected','no','TriggerType',0),'EnablePortSelected','yes','UserCoding',struct('Selected','no','InterfaceFile','UserEncodingFile','FcnName','UserEncodeFcn','InportSelected','no','InportWidth',1,'OutportSelected','no','OutportWidth',1),'TerminationMsg',struct('Selected','no','Byte0','0x00','Byte1','0x00','Byte2','0x00','Byte3','0x00','Byte4','0x00','Byte5','0x00','Byte6','0x00','Byte7','0x00'),'InitialMsg',struct('Selected','no','Byte0','0x00','Byte1','0x00','Byte2','0x00','Byte3','0x00','Byte4','0x00','Byte5','0x00','Byte6','0x00','Byte7','0x00'),'BoardType','DS1','BoardNo',3,'ControllerNo',1),'OFF',[]}},'TLCFileName',{{'rtican_tx_message','OFF',[]}})  RTISFcnParameters=struct('SFcnRTICANMessage','struct','TLCFileName','char')  RTIBlockParaDefault=struct('BoardTypeNo',4302,'BoardNo',1,'ChannelNo',1,'Parameters',struct('DataFileSupport',struct('DataFileSelectedMaster',0,'DataFileSelectedLocal',0,'DataFileName','','DataFileDate','','SelectedFile',['<no file selected>']),'Options',struct('StatusSelected',1,'TimeSelected',1,'DeltaTimeSelected',1,'DelayTimeSelected',1,'DelayTimeTXCommandSelected',0,'EncodeSetUnusedBitsToOne',0,'EnableMsgLoopback',0,'TriggerPort',struct('Selected',0,'TriggerType','rising'),'EnablePortSelected',0,'SignalOnPortnameSelected',1,'UserCoding',struct('Selected',0,'InterfaceFile','UserEncodingFile','FcnName','UserEncodeFcn','InportSelected',0,'InportWidth',1,'OutportSelected',0,'OutportWidth',1),'TerminationMsg',struct('Selected',0,'Byte0_7','0'),'InitialMsg',struct('Selected',0,'Byte0_7','0')),'Message',struct('MsgOnBlocknameSelected',0,'MsgName',['TX Message'],'MsgIdFormat',0,'MsgId',100,'MsgLength',8,'NumSignals',1,'SampleTime',-1,'StartTime',struct('Selected',0,'Value',0),'AutoRepeatTime',struct('Selected',0,'Value',0.1),'Timeout',struct('Selected',0,'Value',0.1),'DelayTime',struct('Selected',0,'Value',0.1),'Signal',struct('SgnName',['TX signal'],'SgnStartBit',0,'SgnLength',8,'SgnType',0,'ModeValue',-1,'DataType',0,'SLDataType','SS_DOUBLE','ByteLayout',0,'Factor',1,'Offset',0,'Min',0,'Max',255,'SgnComment',{{}},'SgnUnit',''),'MsgIdNumFormat',0,'MsgComment',{{''}}),'Version',1.2,'general',struct('isFromLib',1)),'GroupId',struct('Group',{{'RTICAN'}},'No',1,'Behavior',{{'NAMECHANGE'}},'BlockType',{{'SINK'}},'NameChangeFlag',0),'SFcnRTICANMessage',struct('MsgType','TX','MsgName',['TX Message'],'MsgIdFormat','STD','MsgId',100,'MsgLength',2,'NumSignals',1,'SampleTime',-1,'StartTime',struct('Selected','no','Value',0),'AutoRepeatTime',struct('Selected','no','Value',0.1),'Timeout',struct('Selected','no','Value',0.1),'DelayTime',struct('Selected','no','Value',0.1),'Signal',struct('SgnName',['TX signal'],'SgnStartBit',0,'SgnLength',8,'SgnType','standard','ModeValue',-1,'DataType',['unsigned int'],'ByteLayout',['little endian'],'SLDataType','SS_DOUBLE','Factor',1,'Offset',0),'StatusSelected','yes','TimeSelected','yes','DeltaTimeSelected','yes','DelayTimeSelected','yes','EnablePortSelected','no','EnableMsgLoopback','no','DelayTimeTXCommandSelected','no','EncodeSetUnusedBitsToOne','no','UserCoding',struct('Selected','no','InterfaceFile','UserDecodingFile','FcnName','UserDecodeFcn','InportSelected','no','InportWidth',1,'OutportSelected','no','OutportWidth',1),'TerminationMsg',struct('Selected','no','Byte0','0x00','Byte1','0x00','Byte2','0x00','Byte3','0x00','Byte4','0x00','Byte5','0x00','Byte6','0x00','Byte7','0x00'),'InitialMsg',struct('Selected','no','Byte0','0x00','Byte1','0x00','Byte2','0x00','Byte3','0x00','Byte4','0x00','Byte5','0x00','Byte6','0x00','Byte7','0x00'),'TriggerPort',struct('Selected','no','TriggerType','rising'),'BoardType','DS4302','BoardNo',1,'ControllerNo',1,'SFcnPortType','Scalar'),'TLCFileName','rtican_tx_message')
      settings: AttributesFormatString=Group Id: RTICAN5\n  SourceProductName=dSPACE RTI CAN Blockset
  Terminator{,1..3} (4 alike) : Terminator
      settings: InitFcn=|
      | try
      |    MBDS_BlockCallback('Update', gcb);
      | end
  wires:
  Bus Selector/17 -> CCVS1_00/17  "<EngIdleIncrementSwitch>"
  Bus Selector/20 -> CCVS1_00/20  "<EngShutdownOverrideSwitch>"
  Bus Selector/4 -> CCVS1_00/4  "<ParkBrakeReleaseInhibitRq>"
  Bus Selector/6 -> CCVS1_00/6  "<CruiseCtrlActive>"
  Bus Selector/14 -> CCVS1_00/14  "<CruiseCtrlSetSpeed>"
  Bus Selector/11 -> CCVS1_00/11  "<CruiseCtrlCoastSwitch>"
  Bus Selector/3 -> CCVS1_00/3  "<CruiseCtrlPauseSwitch>"
  Bus Selector/2 -> CCVS1_00/2  "<ParkingBrakeSwitch>"
  Bus Selector/16 -> CCVS1_00/16  "<CruiseCtrlStates>"
  Bus Selector/5 -> CCVS1_00/5  "<WheelBasedVehicleSpeed>"
  Bus Selector/8 -> CCVS1_00/8  "<BrakeSwitch>"
  Bus Selector/13 -> CCVS1_00/13  "<CruiseCtrlAccelerateSwitch>"
  Bus Selector/10 -> CCVS1_00/10  "<CruiseCtrlSetSwitch>"
  Bus Selector/7 -> CCVS1_00/7  "<CruiseCtrlEnableSwitch>"
  Bus Selector/9 -> CCVS1_00/9  "<ClutchSwitch>"
  Bus Selector/18 -> CCVS1_00/18  "<EngIdleDecrementSwitch>"
  Bus Selector/12 -> CCVS1_00/12  "<CruiseCtrlResumeSwitch>"
  Bus Selector/19 -> CCVS1_00/19  "<EngTestModeSwitch>"
  Bus Selector/15 -> CCVS1_00/15  "<PTOGovernorState>"
  Bus Selector/1 -> CCVS1_00/1  "<TwoSpeedAxleSwitch>"
  Enable/1 -> CCVS1_00/Enable
  CCVS1_00/1 -> Terminator/1
  CCVS1_00/3 -> Terminator2/1
  CCVS1_00/4 -> Terminator3/1
  CCVS1_00/2 -> Terminator1/1
  Data/1 -> Bus Selector/1
